simulink model "14_bus"  (R2024a)
settings: Solver=VariableStepAuto  StartTime=0.0  StopTime=1  RelTol=1e-3
undefined symbols (not defined in the file): D1, Delta
libraries: spsRMSLib x186, simulink_extras x171, spsThreePhaseVIMeasurementLib x94, spsThreePhaseBreakerLib x62, spsThreePhaseSeriesRLCBranchLib x20, spsThreePhaseSeriesRLCLoadLib x12, spsThreePhaseSourceLib x5, spsLoadFlowBusLib x5, spsStairGeneratorLib x5, spsThreePhaseTransformerTwoWindingsLib x5, spsThreePhaseFaultLib x5, sps_lib x1
(part 1 of 6)
settings Model: VariantFading=off  Creator=kedar  LastModifiedBy=kedar

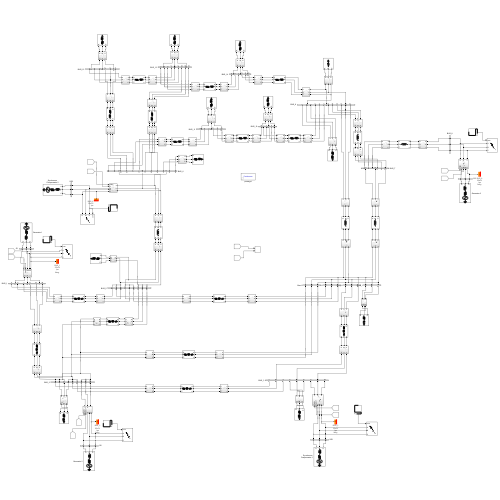
[thumbnail: Simulink's stored preview of the top-level diagram]
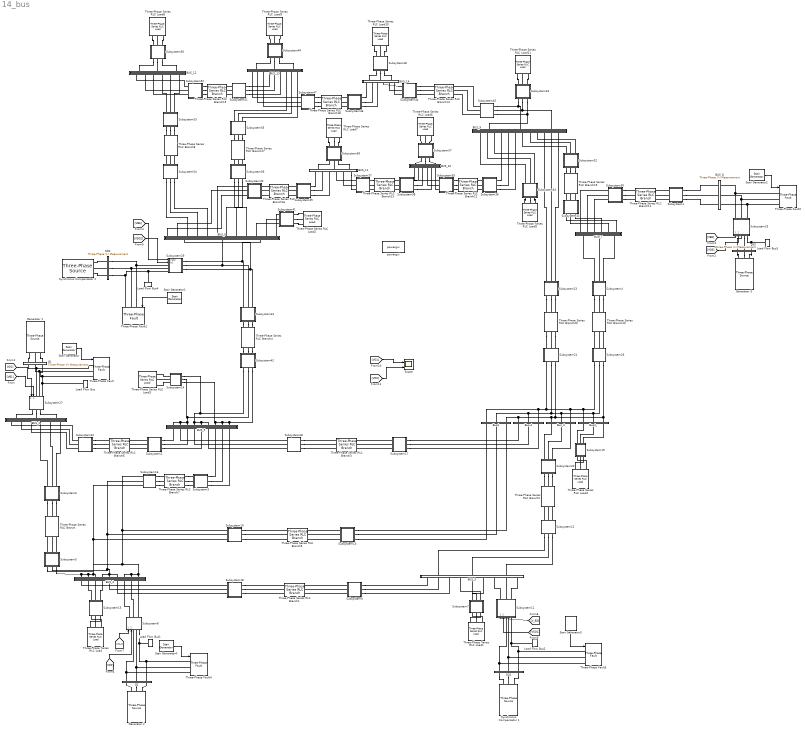
== system 14_bus ==
  BUS_1 : Subsystem
  BUS_10 : Subsystem
  BUS_11 : Subsystem
  BUS_12 : Subsystem
  BUS_13 : Subsystem
  BUS_14 : Subsystem
  BUS_2 : Subsystem
  BUS_3 : Subsystem
  BUS_5 : Subsystem
  BUS_6 : Subsystem
  BUS_7 : Subsystem
  BUS_8 : spsThreePhaseVIMeasurementLib/Three-Phase V-I Measurement  VoltageMeasurement=phase-to-ground  SetLabelV=on  LabelV=VB8  Vpu=off  VpuLL=off  CurrentMeasurement=yes  SetLabelI=on  LabelI=IB8  Ipu=off  Pbase=100e6  Vbase=0.95  OutputType=Complex  PhasorSimulation=off  PSBequivalent=0
  BUS_9 : Subsystem
  Bus-4 : spsThreePhaseVIMeasurementLib/Three-Phase V-I Measurement  VoltageMeasurement=phase-to-ground  SetLabelV=on  LabelV=VB4  Vpu=off  VpuLL=off  CurrentMeasurement=yes  SetLabelI=on  LabelI=IB4  Ipu=off  Pbase=100e6  Vbase=0.95  OutputType=Complex  PhasorSimulation=off  PSBequivalent=0
  Bus4 : spsThreePhaseVIMeasurementLib/Three-Phase V-I Measurement  VoltageMeasurement=phase-to-ground  SetLabelV=on  LabelV=VB_4  Vpu=off  VpuLL=off  CurrentMeasurement=yes  SetLabelI=on  LabelI=IB_4  Ipu=off  Pbase=100e6  Vbase=0.95  OutputType=Complex  PhasorSimulation=off  PSBequivalent=0
  Bus4_ : spsThreePhaseVIMeasurementLib/Three-Phase V-I Measurement  VoltageMeasurement=phase-to-ground  SetLabelV=on  LabelV=VB4_  Vpu=off  VpuLL=off  CurrentMeasurement=yes  SetLabelI=on  LabelI=IB4_  Ipu=off  Pbase=100e6  Vbase=0.95  OutputType=Complex  PhasorSimulation=off  PSBequivalent=0
  Bus_4 : spsThreePhaseVIMeasurementLib/Three-Phase V-I Measurement  VoltageMeasurement=phase-to-ground  SetLabelV=on  LabelV=V_B4  Vpu=off  VpuLL=off  CurrentMeasurement=yes  SetLabelI=on  LabelI=I_B4  Ipu=off  Pbase=100e6  Vbase=0.95  OutputType=Complex  PhasorSimulation=off  PSBequivalent=0
  G1 : spsThreePhaseVIMeasurementLib/Three-Phase V-I Measurement  VoltageMeasurement=phase-to-ground  SetLabelV=on  LabelV=VG1  Vpu=off  VpuLL=off  CurrentMeasurement=yes  SetLabelI=on  LabelI=IG1  Ipu=off  Pbase=100e6  Vbase=25e3  OutputType=Complex  PhasorSimulation=off  PSBequivalent=0
  G2 : spsThreePhaseVIMeasurementLib/Three-Phase V-I Measurement  VoltageMeasurement=phase-to-ground  SetLabelV=on  LabelV=VG2  Vpu=off  VpuLL=off  CurrentMeasurement=yes  SetLabelI=on  LabelI=IG2  Ipu=off  Pbase=100e6  Vbase=500e3  OutputType=Complex  PhasorSimulation=off  PSBequivalent=0
  G3 : spsThreePhaseVIMeasurementLib/Three-Phase V-I Measurement  VoltageMeasurement=phase-to-ground  SetLabelV=on  LabelV=VG3  Vpu=off  VpuLL=off  CurrentMeasurement=yes  SetLabelI=on  LabelI=IG3  Ipu=off  Pbase=100e6  Vbase=500e3  OutputType=Complex  PhasorSimulation=off  PSBequivalent=0
  Generator 1 : spsThreePhaseSourceLib/Three-Phase Source  InternalConnection=Yg  VoltagePhases=off  Voltage=25e3*1.060  PhaseAngle=0  Voltage_phases=[25e3 25e3 25e3]/sqrt(3)  PhaseAngles_phases=[0 -120 +120]  Frequency=50  NonIdealSource=on  SpecifyImpedance=on  Resistance=0.8929  Inductance=16.58e-3  ShortCircuitLevel=100e6  BaseVoltage=25e3  XRratio=7  BusType=swing  Pref=40e3  Qref=-40e3  Prefabc=[10e3, 10e3, 10e3]  Qrefabc=[0, 0, 0]  Qmin=-inf  Qmax=inf
  Generator 2 : spsThreePhaseSourceLib/Three-Phase Source  InternalConnection=Yg  VoltagePhases=off  Voltage=25e3*1.045  PhaseAngle=0  Voltage_phases=[25e3 25e3 25e3]/sqrt(3)  PhaseAngles_phases=[0 -120 +120]  Frequency=50  NonIdealSource=on  SpecifyImpedance=off  Resistance=0.8929  Inductance=16.58e-3  ShortCircuitLevel=100e6  BaseVoltage=25e3  XRratio=7  BusType=PV  Pref=232e3  Qref=0  Prefabc=[10e3, 10e3, 10e3]  Qrefabc=[0, 0, 0]  Qmin=-40e3  Qmax=50e3
  Generator 3 : spsThreePhaseSourceLib/Three-Phase Source  InternalConnection=Yg  VoltagePhases=off  Voltage=25e3*1.09  PhaseAngle=0  Voltage_phases=[25e3 25e3 25e3]/sqrt(3)  PhaseAngles_phases=[0 -120 +120]  Frequency=50  NonIdealSource=on  SpecifyImpedance=off  Resistance=0.8929  Inductance=16.58e-3  ShortCircuitLevel=100e6  BaseVoltage=25e3  XRratio=7  BusType=PQ  Pref=0  Qref=0  Prefabc=[10e3, 10e3, 10e3]  Qrefabc=[0, 0, 0]  Qmin=-6e3  Qmax=24e3
  Load Flow Bus : spsLoadFlowBusLib/Load Flow Bus  LConnTagsString=a  Phases=single  Connectors=on one side  ID=BUS_1  Vbase=25e3  Vref=1.06  Vangle=0  VLF=1  VLFb=1  VLFc=1  angleLF=0  angleLFb=0  angleLFc=0
  Load Flow Bus1 : spsLoadFlowBusLib/Load Flow Bus  LConnTagsString=a  Phases=single  Connectors=on one side  ID=BUS_2  Vbase=25e3  Vref=1.045  Vangle=0  VLF=1  VLFb=1  VLFc=1  angleLF=0  angleLFb=0  angleLFc=0
  Load Flow Bus2 : spsLoadFlowBusLib/Load Flow Bus  LConnTagsString=a  Phases=single  Connectors=on one side  ID=BUS_3  Vbase=25e3  Vref=1.01  Vangle=0  VLF=1  VLFb=1  VLFc=1  angleLF=0  angleLFb=0  angleLFc=0
  Load Flow Bus3 : spsLoadFlowBusLib/Load Flow Bus  LConnTagsString=a  Phases=single  Connectors=on one side  ID=BUS_8  Vbase=25e3  Vref=1.09  Vangle=0  VLF=1  VLFb=1  VLFc=1  angleLF=0  angleLFb=0  angleLFc=0
  Load Flow Bus4 : spsLoadFlowBusLib/Load Flow Bus  LConnTagsString=a  Phases=single  Connectors=on one side  ID=BUS_6  Vbase=25e3  Vref=1.07  Vangle=0  VLF=1  VLFb=1  VLFc=1  angleLF=0  angleLFb=0  angleLFc=0
  SG1 : spsThreePhaseVIMeasurementLib/Three-Phase V-I Measurement  VoltageMeasurement=phase-to-ground  SetLabelV=on  LabelV=VSG1  Vpu=off  VpuLL=off  CurrentMeasurement=yes  SetLabelI=on  LabelI=ISG1  Ipu=off  Pbase=100e6  Vbase=500e3  OutputType=Complex  PhasorSimulation=off  PSBequivalent=0
  SG2 : spsThreePhaseVIMeasurementLib/Three-Phase V-I Measurement  VoltageMeasurement=phase-to-ground  SetLabelV=on  LabelV=VSG2  Vpu=off  VpuLL=off  CurrentMeasurement=yes  SetLabelI=on  LabelI=ISG2  Ipu=off  Pbase=100e6  Vbase=500e3  OutputType=Complex  PhasorSimulation=off  PSBequivalent=0
  Scope : Scope  NumInputPorts=2
  Stair Generator{,1..4} (5 alike) : spsStairGeneratorLib/Stair Generator  t=[0, 1, 3, 3.5]  e=[1, -1, 2.5, 0]  Ts=0
  Subsystem1 : Subsystem
  Subsystem10 : Subsystem
  Subsystem11 : Subsystem
  Subsystem12 : Subsystem
  Subsystem13 : Subsystem
  Subsystem14 : Subsystem
  Subsystem15 : Subsystem
  Subsystem16 : Subsystem
  Subsystem17 : Subsystem
  Subsystem18 : Subsystem
  Subsystem19 : Subsystem
  Subsystem2 : Subsystem
  Subsystem20 : Subsystem
  Subsystem21 : Subsystem
  Subsystem22 : Subsystem
  Subsystem23 : Subsystem
  Subsystem25 : Subsystem
  Subsystem26 : Subsystem
  Subsystem27 : Subsystem
  Subsystem28 : Subsystem
  Subsystem29 : Subsystem
  Subsystem3 : Subsystem
  Subsystem30 : Subsystem
  Subsystem31 : Subsystem
  Subsystem32 : Subsystem
  Subsystem33 : Subsystem
  Subsystem34 : Subsystem
  Subsystem35 : Subsystem
  Subsystem36 : Subsystem
  Subsystem37 : Subsystem
  Subsystem38 : Subsystem
  Subsystem39 : Subsystem
  Subsystem4 : Subsystem
  Subsystem40 : Subsystem
  Subsystem41 : Subsystem
  Subsystem42 : Subsystem
  Subsystem43 : Subsystem
  Subsystem44 : Subsystem
  Subsystem45 : Subsystem
  Subsystem46 : Subsystem
  Subsystem47 : Subsystem
  Subsystem48 : Subsystem
  Subsystem49 : Subsystem
  Subsystem5 : Subsystem
  Subsystem50 : Subsystem
  Subsystem51 : Subsystem
  Subsystem52 : Subsystem
  Subsystem53 : Subsystem
  Subsystem54 : Subsystem
  Subsystem55 : Subsystem
  Subsystem56 : Subsystem
  Subsystem57 : Subsystem
  Subsystem58 : Subsystem
  Subsystem6 : Subsystem
  Subsystem7 : Subsystem
  Subsystem8 : Subsystem
  Subsystem9 : Subsystem
  Synchronus Compensator 1 : spsThreePhaseSourceLib/Three-Phase Source  InternalConnection=Yg  VoltagePhases=off  Voltage=25e3*1.01  PhaseAngle=0  Voltage_phases=[25e3 25e3 25e3]/sqrt(3)  PhaseAngles_phases=[0 -120 +120]  Frequency=50  NonIdealSource=on  SpecifyImpedance=off  Resistance=0.8929  Inductance=16.58e-3  ShortCircuitLevel=100e6  BaseVoltage=25e3  XRratio=7  BusType=PV  Pref=0  Qref=0  Prefabc=[10e3, 10e3, 10e3]  Qrefabc=[0, 0, 0]  Qmin=0  Qmax=50e3
  Synchronus Compensator 2 : spsThreePhaseSourceLib/Three-Phase Source  InternalConnection=Yg  VoltagePhases=off  Voltage=25e3*1.07  PhaseAngle=0  Voltage_phases=[25e3 25e3 25e3]/sqrt(3)  PhaseAngles_phases=[0 -120 +120]  Frequency=50  NonIdealSource=on  SpecifyImpedance=off  Resistance=0.8929  Inductance=16.58e-3  ShortCircuitLevel=100e6  BaseVoltage=25e3  XRratio=7  BusType=PV  Pref=0  Qref=0  Prefabc=[10e3, 10e3, 10e3]  Qrefabc=[0, 0, 0]  Qmin=-6e3  Qmax=24e3
  Three-Phase Series RLC Branch : spsThreePhaseSeriesRLCBranchLib/Three-Phase Series RLC Branch  LConnTagsString=A|B|C  RConnTagsString=A|B|C  BranchType=RLC  Resistance=1.94e-2  Inductance=0.05917/(2*pi*50)  Capacitance=1/0.0528/(2*pi*50)  Measurements=None
  Three-Phase Series RLC Branch1 : spsThreePhaseSeriesRLCBranchLib/Three-Phase Series RLC Branch  LConnTagsString=A|B|C  RConnTagsString=A|B|C  BranchType=RLC  Resistance=0.04699  Inductance=0.19797/(2*pi*50)  Capacitance=1/0.0374/(2*pi*50)  Measurements=None
  Three-Phase Series RLC Branch10 : spsThreePhaseSeriesRLCBranchLib/Three-Phase Series RLC Branch  LConnTagsString=A|B|C  RConnTagsString=A|B|C  BranchType=L  Resistance=0  Inductance=0.20912/(2*pi*50)  Capacitance=0  Measurements=None
  Three-Phase Series RLC Branch11 : spsThreePhaseSeriesRLCBranchLib/Three-Phase Series RLC Branch  LConnTagsString=A|B|C  RConnTagsString=A|B|C  BranchType=L  Resistance=0  Inductance=0.17615/(2*pi*50)  Capacitance=0  Measurements=None
  Three-Phase Series RLC Branch12 : spsThreePhaseSeriesRLCBranchLib/Three-Phase Series RLC Branch  LConnTagsString=A|B|C  RConnTagsString=A|B|C  BranchType=RL  Resistance=0.03181  Inductance=0.0845/(2*pi*50)  Capacitance=1e-6  Measurements=None
  Three-Phase Series RLC Branch13 : spsThreePhaseSeriesRLCBranchLib/Three-Phase Series RLC Branch  LConnTagsString=A|B|C  RConnTagsString=A|B|C  BranchType=RL  Resistance=0.08205  Inductance=0.19207/(2*pi*50)  Capacitance=1e-6  Measurements=None
  Three-Phase Series RLC Branch14 : spsThreePhaseSeriesRLCBranchLib/Three-Phase Series RLC Branch  LConnTagsString=A|B|C  RConnTagsString=A|B|C  BranchType=RL  Resistance=0.12711  Inductance=0.27038/(2*pi*50)  Capacitance=1e-6  Measurements=None
  Three-Phase Series RLC Branch15 : spsThreePhaseSeriesRLCBranchLib/Three-Phase Series RLC Branch  LConnTagsString=A|B|C  RConnTagsString=A|B|C  BranchType=RL  Resistance=0.22092  Inductance=0.19988/(2*pi*50)  Capacitance=1e-6  Measurements=None
  Three-Phase Series RLC Branch16 : spsThreePhaseSeriesRLCBranchLib/Three-Phase Series RLC Branch  LConnTagsString=A|B|C  RConnTagsString=A|B|C  BranchType=RL  Resistance=0.09498  Inductance=0.1989/(2*pi*50)  Capacitance=1e-6  Measurements=None
  Three-Phase Series RLC Branch17 : spsThreePhaseSeriesRLCBranchLib/Three-Phase Series RLC Branch  LConnTagsString=A|B|C  RConnTagsString=A|B|C  BranchType=RL  Resistance=0.06615  Inductance=0.13027/(2*pi*50)  Capacitance=1e-6  Measurements=None
  Three-Phase Series RLC Branch18 : spsThreePhaseSeriesRLCBranchLib/Three-Phase Series RLC Branch  LConnTagsString=A|B|C  RConnTagsString=A|B|C  BranchType=RL  Resistance=0.17093  Inductance=0.34802/(2*pi*50)  Capacitance=1e-6  Measurements=None
  Three-Phase Series RLC Branch19 : spsThreePhaseSeriesRLCBranchLib/Three-Phase Series RLC Branch  LConnTagsString=A|B|C  RConnTagsString=A|B|C  BranchType=L  Resistance=1  Inductance=0.11001/(2*pi*50)  Capacitance=1e-6  Measurements=None
  Three-Phase Series RLC Branch2 : spsThreePhaseSeriesRLCBranchLib/Three-Phase Series RLC Branch  LConnTagsString=A|B|C  RConnTagsString=A|B|C  BranchType=RLC  Resistance=0.06701  Inductance=0.17103/(2*pi*50)  Capacitance=1/0.0346/(2*pi*50)  Measurements=None
  Three-Phase Series RLC Branch20 : spsThreePhaseSeriesRLCBranchLib/Three-Phase Series RLC Branch  LConnTagsString=A|B|C  RConnTagsString=A|B|C  BranchType=L  Resistance=1  Inductance=0.55618/(2*pi*50)  Capacitance=1e-6  Measurements=None
  Three-Phase Series RLC Branch3 : spsThreePhaseSeriesRLCBranchLib/Three-Phase Series RLC Branch  LConnTagsString=A|B|C  RConnTagsString=A|B|C  BranchType=RLC  Resistance=0.01335  Inductance=0.04211/(2*pi*50)  Capacitance=1/0.0128/(2*pi*50)  Measurements=None
  Three-Phase Series RLC Branch4 : spsThreePhaseSeriesRLCBranchLib/Three-Phase Series RLC Branch  LConnTagsString=A|B|C  RConnTagsString=A|B|C  BranchType=L  Resistance=0  Inductance=0.25202/(2*pi*50)  Capacitance=0  Measurements=None
  Three-Phase Series RLC Branch5 : spsThreePhaseSeriesRLCBranchLib/Three-Phase Series RLC Branch  LConnTagsString=A|B|C  RConnTagsString=A|B|C  BranchType=RLC  Resistance=0.05811  Inductance=0.17632/(2*pi*50)  Capacitance=1/0.0492/(2*pi*50)  Measurements=None
  Three-Phase Series RLC Branch6 : spsThreePhaseSeriesRLCBranchLib/Three-Phase Series RLC Branch  LConnTagsString=A|B|C  RConnTagsString=A|B|C  BranchType=RLC  Resistance=0.05403  Inductance=0.22304/(2*pi*50)  Capacitance=1/0.0438/(2*pi*50)  Measurements=None
  Three-Phase Series RLC Branch7 : spsThreePhaseSeriesRLCBranchLib/Three-Phase Series RLC Branch  LConnTagsString=A|B|C  RConnTagsString=A|B|C  BranchType=RLC  Resistance=0.05695  Inductance=0.17388/(2*pi*50)  Capacitance=1/0.034/(2*pi*50)  Measurements=None
  Three-Phase Series RLC Branch8 : spsThreePhaseSeriesRLCBranchLib/Three-Phase Series RLC Branch  LConnTagsString=A|B|C  RConnTagsString=A|B|C  BranchType=RL  Resistance=0.12291  Inductance=0.25581/(2*pi*50)  Capacitance=1e-6  Measurements=None
  Three-Phase Series RLC Load : spsThreePhaseSeriesRLCLoadLib/Three-Phase Series RLC Load  LConnTagsString=A|B|C  Configuration=Y (grounded)  NominalVoltage=25e3*1.045  Vabc=[1e3 1e3 1e3]  Vabcp=[1e3 1e3 1e3]  NominalFrequency=50  UnbalancedPower=off  ActivePower=21.7e3  InductivePower=12.7e3  CapacitivePower=0  Pabc=[10e3 9e3 11e3]  QLabc=[100 90 110]  QCabc=[100 90 110]  Pabcp=[10e3 9e3 11e3]  QLabcp=[100 90 110]  QCabcp=[100 90 110]  Measurements=None  LoadType=constant Z
  Three-Phase Series RLC Load1 : spsThreePhaseSeriesRLCLoadLib/Three-Phase Series RLC Load  LConnTagsString=A|B|C  Configuration=Y (grounded)  NominalVoltage=25e3*1.01  Vabc=[1e3 1e3 1e3]  Vabcp=[1e3 1e3 1e3]  NominalFrequency=50  UnbalancedPower=off  ActivePower=94.2e3  InductivePower=19.1e3  CapacitivePower=0  Pabc=[10e3 9e3 11e3]  QLabc=[100 90 110]  QCabc=[100 90 110]  Pabcp=[10e3 9e3 11e3]  QLabcp=[100 90 110]  QCabcp=[100 90 110]  Measurements=None  LoadType=constant Z
  Three-Phase Series RLC Load10 : spsThreePhaseSeriesRLCLoadLib/Three-Phase Series RLC Load  LConnTagsString=A|B|C  Configuration=Y (grounded)  NominalVoltage=25e3  Vabc=[1e3 1e3 1e3]  Vabcp=[1e3 1e3 1e3]  NominalFrequency=50  UnbalancedPower=off  ActivePower=14.9e3  InductivePower=5e3  CapacitivePower=0  Pabc=[10e3 9e3 11e3]  QLabc=[100 90 110]  QCabc=[100 90 110]  Pabcp=[10e3 9e3 11e3]  QLabcp=[100 90 110]  QCabcp=[100 90 110]  Measurements=None  LoadType=constant Z
  Three-Phase Series RLC Load11 : spsThreePhaseSeriesRLCLoadLib/Three-Phase Series RLC Load  LConnTagsString=A|B|C  Configuration=Y (grounded)  NominalVoltage=25e3  Vabc=[1e3 1e3 1e3]  Vabcp=[1e3 1e3 1e3]  NominalFrequency=50  UnbalancedPower=off  ActivePower=0  InductivePower=0  CapacitivePower=25e6  Pabc=[10e3 9e3 11e3]  QLabc=[100 90 110]  QCabc=[100 90 110]  Pabcp=[10e3 9e3 11e3]  QLabcp=[100 90 110]  QCabcp=[100 90 110]  Measurements=None  LoadType=constant Z
  Three-Phase Series RLC Load2 : spsThreePhaseSeriesRLCLoadLib/Three-Phase Series RLC Load  LConnTagsString=A|B|C  Configuration=Y (grounded)  NominalVoltage=25e3*1.07  Vabc=[1e3 1e3 1e3]  Vabcp=[1e3 1e3 1e3]  NominalFrequency=50  UnbalancedPower=off  ActivePower=11.2e3  InductivePower=7.5e3  CapacitivePower=0  Pabc=[10e3 9e3 11e3]  QLabc=[100 90 110]  QCabc=[100 90 110]  Pabcp=[10e3 9e3 11e3]  QLabcp=[100 90 110]  QCabcp=[100 90 110]  Measurements=None  LoadType=constant Z
  Three-Phase Series RLC Load3 : spsThreePhaseSeriesRLCLoadLib/Three-Phase Series RLC Load  LConnTagsString=A|B|C  Configuration=Y (grounded)  NominalVoltage=25e3  Vabc=[1e3 1e3 1e3]  Vabcp=[1e3 1e3 1e3]  NominalFrequency=50  UnbalancedPower=off  ActivePower=7.6e3  InductivePower=1.6e3  CapacitivePower=0  Pabc=[10e3 9e3 11e3]  QLabc=[100 90 110]  QCabc=[100 90 110]  Pabcp=[10e3 9e3 11e3]  QLabcp=[100 90 110]  QCabcp=[100 90 110]  Measurements=None  LoadType=constant Z
  Three-Phase Series RLC Load4 : spsThreePhaseSeriesRLCLoadLib/Three-Phase Series RLC Load  LConnTagsString=A|B|C  Configuration=Y (grounded)  NominalVoltage=25e3  Vabc=[1e3 1e3 1e3]  Vabcp=[1e3 1e3 1e3]  NominalFrequency=50  UnbalancedPower=off  ActivePower=47.8e3  InductivePower=0  CapacitivePower=3.9e3  Pabc=[10e3 9e3 11e3]  QLabc=[100 90 110]  QCabc=[100 90 110]  Pabcp=[10e3 9e3 11e3]  QLabcp=[100 90 110]  QCabcp=[100 90 110]  Measurements=None  LoadType=constant Z
  Three-Phase Series RLC Load5 : spsThreePhaseSeriesRLCLoadLib/Three-Phase Series RLC Load  LConnTagsString=A|B|C  Configuration=Y (grounded)  NominalVoltage=25e3*1.07  Vabc=[1e3 1e3 1e3]  Vabcp=[1e3 1e3 1e3]  NominalFrequency=50  UnbalancedPower=off  ActivePower=29.5e3  InductivePower=16.6e3  CapacitivePower=0  Pabc=[10e3 9e3 11e3]  QLabc=[100 90 110]  QCabc=[100 90 110]  Pabcp=[10e3 9e3 11e3]  QLabcp=[100 90 110]  QCabcp=[100 90 110]  Measurements=None  LoadType=constant Z
  Three-Phase Series RLC Load6 : spsThreePhaseSeriesRLCLoadLib/Three-Phase Series RLC Load  LConnTagsString=A|B|C  Configuration=Y (grounded)  NominalVoltage=25e3*1.09  Vabc=[1e3 1e3 1e3]  Vabcp=[1e3 1e3 1e3]  NominalFrequency=50  UnbalancedPower=off  ActivePower=9e3  InductivePower=5.8e3  CapacitivePower=0  Pabc=[10e3 9e3 11e3]  QLabc=[100 90 110]  QCabc=[100 90 110]  Pabcp=[10e3 9e3 11e3]  QLabcp=[100 90 110]  QCabcp=[100 90 110]  Measurements=None  LoadType=constant Z
  Three-Phase Series RLC Load7 : spsThreePhaseSeriesRLCLoadLib/Three-Phase Series RLC Load  LConnTagsString=A|B|C  Configuration=Y (grounded)  NominalVoltage=25e3  Vabc=[1e3 1e3 1e3]  Vabcp=[1e3 1e3 1e3]  NominalFrequency=50  UnbalancedPower=off  ActivePower=3.5e3  InductivePower=1.8e3  CapacitivePower=0  Pabc=[10e3 9e3 11e3]  QLabc=[100 90 110]  QCabc=[100 90 110]  Pabcp=[10e3 9e3 11e3]  QLabcp=[100 90 110]  QCabcp=[100 90 110]  Measurements=None  LoadType=constant Z
  Three-Phase Series RLC Load8 : spsThreePhaseSeriesRLCLoadLib/Three-Phase Series RLC Load  LConnTagsString=A|B|C  Configuration=Y (grounded)  NominalVoltage=25e3  Vabc=[1e3 1e3 1e3]  Vabcp=[1e3 1e3 1e3]  NominalFrequency=50  UnbalancedPower=off  ActivePower=6.1e3  InductivePower=1.6e3  CapacitivePower=0  Pabc=[10e3 9e3 11e3]  QLabc=[100 90 110]  QCabc=[100 90 110]  Pabcp=[10e3 9e3 11e3]  QLabcp=[100 90 110]  QCabcp=[100 90 110]  Measurements=None  LoadType=constant Z
  Three-Phase Series RLC Load9 : spsThreePhaseSeriesRLCLoadLib/Three-Phase Series RLC Load  LConnTagsString=A|B|C  Configuration=Y (grounded)  NominalVoltage=25e3  Vabc=[1e3 1e3 1e3]  Vabcp=[1e3 1e3 1e3]  NominalFrequency=50  UnbalancedPower=off  ActivePower=13.8e3  InductivePower=5.8e3  CapacitivePower=0  Pabc=[10e3 9e3 11e3]  QLabc=[100 90 110]  QCabc=[100 90 110]  Pabcp=[10e3 9e3 11e3]  QLabcp=[100 90 110]  QCabcp=[100 90 110]  Measurements=None  LoadType=constant Z
  Three-Phase Fault{,1..4} (5 alike) : spsThreePhaseFaultLib/Three-Phase Fault  InitialStates=0  FaultA=off  FaultB=off  FaultC=off  GroundFault=off  SwitchTimes="[1/60  5/60]"  External=on  SwitchStatus=NaN  FaultResistance=0.001  GroundResistance=0.01  SnubberResistance=1e6  SnubberCapacitance=inf  Measurements=None
  powergui : sps_lib/powergui  Priority=1  SimulationMode=Continuous  SampleTime=50e-6  frequency=60  Iterations=50  frequencyindice=50  Pbase=100e6  ErrMax=1e-4  UnitsV=kV  UnitsW=MW  buscounter=0  FunctionMessages=off  echomessages=off  EnableUseOfTLC=off  CurrentSourceSwitches=off  DisableSnubberDevices=off  DisableRonSwitches=off  DisableVfSwitches=off  DisplayEquations=off  AutomaticDiscreteSolvers=off  SolverType=Tustin/Backward Euler (TBE)  Interpol=off  ExternalGateDelay=off  methode=off  Ts=100  x0status=blocks  SPID=on  SwTol=0  HookPort=off  NonlinearTolerance=1e-4  nMaxIteration=100  ContinueOnMaxIteration=off  RestoreLinks=warning  ResistiveCurrentMeasurement=off  Frange=[0:2:500]  Ylog=off  Xlog=on  ShowGrid=off  save=off  variable=ZData  structure=0  ZoomFFT=off  StartTime=0.0  cycles=1  DisplayStyle=1  fundamental=60  FreqAxis=off  MaxFrequency=1000  frequencyindicesteady=1  RmsSteady=1  display=off
  wires:
  [VB6] -> Subsystem29/1(Vabc)
  [VG2] -> Subsystem8/2(Vabc1)
  [VB1] -> Subsystem27/2(Vabc)
  [IG1] -> Subsystem27/1(In1)
  [VG3] -> Subsystem25/2(In2)
  [VB8] -> Subsystem25/1(Vabc)
  [VSG2] -> Subsystem29/2(In1)
  [VB_2] -> Subsystem8/1(Vabc)
  [V_B3] -> Subsystem11/1(Vabc)
  [VSG1] -> Subsystem11/2(Vabc1)
  [VG1] -> Scope/1
  [VG2] -> Scope/2
  Stair Generator/1 -> Three-Phase Fault/1
  Stair Generator1/1 -> Three-Phase Fault1/1
  Stair Generator2/1 -> Three-Phase Fault2/1
  Stair Generator3/1 -> Three-Phase Fault3/1
  Stair Generator4/1 -> Three-Phase Fault4/1
  connections:
  BUS_2/LConn9 -- BUS_2/LConn8 -- BUS_2/LConn7 -- Subsystem16/RConn1 -- Subsystem10/RConn1 -- Subsystem5/RConn1
  BUS_5/LConn6 -- BUS_5/LConn5 -- Subsystem14/RConn1 -- Subsystem42/RConn1 -- BUS_5/LConn4
  Bus4_/LConn3 -- Subsystem26/RConn3 -- Subsystem21/RConn3 -- Bus4/LConn3 -- Bus-4/LConn1 -- Bus_4/LConn1
  Bus4_/LConn2 -- Subsystem26/RConn2 -- Bus_4/LConn2 -- Subsystem21/RConn2 -- Bus4/LConn2 -- Bus-4/LConn2
  Bus4_/LConn1 -- Subsystem26/RConn1 -- Bus_4/LConn3 -- Subsystem21/RConn1 -- Bus4/LConn1 -- Bus-4/LConn3
  Subsystem33/RConn1 -- Subsystem45/RConn1 -- BUS_9/LConn2
  Subsystem33/RConn3 -- Subsystem45/RConn3 -- BUS_9/LConn1
  Subsystem33/RConn2 -- Subsystem45/RConn2 -- BUS_9/LConn3
  Subsystem42/RConn3 -- BUS_5/LConn9 -- BUS_5/LConn8 -- Subsystem14/RConn3 -- BUS_5/LConn7
  Subsystem14/RConn2 -- Subsystem42/RConn2 -- BUS_5/LConn2 -- BUS_5/LConn1 -- BUS_5/LConn3
  BUS_2/LConn6 -- Subsystem16/RConn2 -- Subsystem10/RConn2 -- Subsystem5/RConn2 -- BUS_2/LConn5 -- BUS_2/LConn4
  Subsystem43/RConn3 -- Subsystem29/RConn3 -- BUS_6/LConn1
  Subsystem43/RConn1 -- BUS_6/LConn3 -- Subsystem29/RConn1
  Subsystem43/RConn2 -- Subsystem29/RConn2 -- BUS_6/LConn2
  G1/LConn2 -- Generator 1/RConn2
  Generator 1/RConn1 -- G1/LConn1
  G2/LConn2 -- Generator 2/RConn2
  Generator 2/RConn1 -- G2/LConn1
  Generator 2/RConn3 -- G2/LConn3
  SG1/LConn1 -- Synchronus Compensator 1/RConn1
  SG1/LConn2 -- Synchronus Compensator 1/RConn2
  SG1/LConn3 -- Synchronus Compensator 1/RConn3
  G3/LConn2 -- Generator 3/RConn2
  G3/LConn1 -- Generator 3/RConn1
  G3/LConn3 -- Generator 3/RConn3
  Subsystem10/LConn1 -- Three-Phase Series RLC Branch5/LConn1
  Subsystem10/LConn2 -- Three-Phase Series RLC Branch5/LConn2
  Subsystem10/LConn3 -- Three-Phase Series RLC Branch5/LConn3
  Subsystem14/LConn1 -- Three-Phase Series RLC Load3/LConn1
  Subsystem14/LConn2 -- Three-Phase Series RLC Load3/LConn2
  Subsystem14/LConn3 -- Three-Phase Series RLC Load3/LConn3
  Subsystem5/RConn3 -- BUS_2/LConn1 -- BUS_2/LConn2 -- BUS_2/LConn3 -- Subsystem16/RConn3 -- Subsystem10/RConn3
  Subsystem3/RConn1 -- BUS_5/RConn7
  Subsystem3/RConn2 -- BUS_5/RConn8
  Subsystem3/RConn3 -- BUS_5/RConn9
  Three-Phase Series RLC Branch7/RConn1 -- Subsystem3/LConn1
  Three-Phase Series RLC Branch7/RConn2 -- Subsystem3/LConn2
  Three-Phase Series RLC Branch7/RConn3 -- Subsystem3/LConn3
  Subsystem16/LConn1 -- Three-Phase Series RLC Branch7/LConn1
  Subsystem16/LConn2 -- Three-Phase Series RLC Branch7/LConn2
  Subsystem16/LConn3 -- Three-Phase Series RLC Branch7/LConn3
  Subsystem15/RConn1 -- BUS_2/RConn2
  Subsystem15/RConn2 -- BUS_2/RConn3
  Subsystem15/RConn3 -- BUS_2/RConn4
  Subsystem8/RConn1 -- BUS_2/RConn7
  Subsystem8/RConn2 -- BUS_2/RConn8
  Subsystem8/RConn3 -- BUS_2/RConn9
  G2/RConn3 -- Subsystem8/LConn1 -- Three-Phase Fault4/LConn3
  G2/RConn2 -- Subsystem8/LConn2 -- Three-Phase Fault4/LConn2
  Subsystem8/LConn3 -- Load Flow Bus1/LConn1 -- G2/RConn1 -- Three-Phase Fault4/LConn1
  Subsystem7/RConn2 -- BUS_3/RConn5
  Subsystem11/RConn1 -- BUS_3/RConn7
  Subsystem11/RConn2 -- BUS_3/RConn8
  Subsystem11/RConn3 -- BUS_3/RConn9
  SG1/RConn3 -- Three-Phase Fault3/LConn3 -- Subsystem11/LConn1
  SG1/RConn2 -- Three-Phase Fault3/LConn2 -- Subsystem11/LConn2
  SG1/RConn1 -- Three-Phase Fault3/LConn1 -- Load Flow Bus2/LConn1 -- Subsystem11/LConn3
  Subsystem19/RConn1 -- Bus4_/RConn1
  Subsystem19/RConn2 -- Bus4_/RConn2
  Subsystem19/RConn3 -- Bus4_/RConn3
  Three-Phase Series RLC Branch20/RConn1 -- Subsystem21/LConn1
  Subsystem21/LConn2 -- Three-Phase Series RLC Branch20/RConn2
  Three-Phase Series RLC Branch20/RConn3 -- Subsystem21/LConn3
  Subsystem23/RConn1 -- BUS_9/RConn10
  Subsystem23/RConn2 -- BUS_9/RConn11
  Subsystem23/RConn3 -- BUS_9/RConn12
  Subsystem23/LConn2 -- Three-Phase Series RLC Branch20/LConn2
  Subsystem26/LConn1 -- Three-Phase Series RLC Branch10/RConn1
  Subsystem26/LConn2 -- Three-Phase Series RLC Branch10/RConn2
  Subsystem26/LConn3 -- Three-Phase Series RLC Branch10/RConn3
  Subsystem25/RConn1 -- BUS_8/RConn1 -- Three-Phase Fault2/LConn1
  Subsystem25/RConn2 -- BUS_8/RConn2 -- Three-Phase Fault2/LConn2
  Subsystem25/RConn3 -- Three-Phase Fault2/LConn3 -- BUS_8/RConn3
  Subsystem25/LConn1 -- G3/RConn1
  Subsystem25/LConn2 -- G3/RConn2
  Subsystem25/LConn3 -- Load Flow Bus3/LConn1 -- G3/RConn3
  G1/RConn1 -- Three-Phase Fault/LConn1 -- Subsystem27/LConn1
  G1/RConn2 -- Three-Phase Fault/LConn2 -- Subsystem27/LConn2
  G1/RConn3 -- Three-Phase Fault/LConn3 -- Load Flow Bus/LConn1 -- Subsystem27/LConn3
  Subsystem30/LConn1 -- Three-Phase Series RLC Branch11/LConn1
  Subsystem30/LConn2 -- Three-Phase Series RLC Branch11/LConn2
  Subsystem30/LConn3 -- Three-Phase Series RLC Branch11/LConn3
  Subsystem30/RConn1 -- BUS_7/RConn1
  Subsystem30/RConn2 -- BUS_7/RConn2
  Subsystem30/RConn3 -- BUS_7/RConn3
  Subsystem1/LConn1 -- Three-Phase Series RLC Branch11/RConn1
  Subsystem1/LConn2 -- Three-Phase Series RLC Branch11/RConn2
  Subsystem1/LConn3 -- Three-Phase Series RLC Branch11/RConn3
  Subsystem1/RConn2 -- BUS_8/LConn2
  Subsystem1/RConn1 -- BUS_8/LConn1
  Subsystem1/RConn3 -- BUS_8/LConn3
  Subsystem31/LConn1 -- Three-Phase Series RLC Branch19/RConn1
  Subsystem31/LConn2 -- Three-Phase Series RLC Branch19/RConn2
  Subsystem31/LConn3 -- Three-Phase Series RLC Branch19/RConn3
  Subsystem31/RConn2 -- BUS_7/RConn5
  Subsystem32/LConn2 -- Three-Phase Series RLC Branch19/LConn2
  Subsystem32/LConn1 -- Three-Phase Series RLC Branch19/LConn1
  Subsystem32/LConn3 -- Three-Phase Series RLC Branch19/LConn3
  Subsystem32/RConn1 -- BUS_9/RConn7
  Subsystem32/RConn2 -- BUS_9/RConn8
  Subsystem32/RConn3 -- BUS_9/RConn9
  Subsystem33/LConn2 -- Three-Phase Series RLC Load11/LConn2
  Three-Phase Series RLC Load11/LConn1 -- Subsystem33/LConn1
  Three-Phase Series RLC Load11/LConn3 -- Subsystem33/LConn3
  Subsystem34/LConn2 -- Three-Phase Series RLC Load5/LConn2
  Subsystem34/LConn1 -- Three-Phase Series RLC Load5/LConn1
  Subsystem34/LConn3 -- Three-Phase Series RLC Load5/LConn3
  Subsystem34/RConn1 -- BUS_9/RConn1
  Subsystem34/RConn2 -- BUS_9/RConn2
  Subsystem34/RConn3 -- BUS_9/RConn3
  Subsystem35/LConn1 -- Three-Phase Series RLC Branch12/LConn1
  Subsystem35/LConn2 -- Three-Phase Series RLC Branch12/LConn2
  Subsystem35/LConn3 -- Three-Phase Series RLC Branch12/LConn3
  Subsystem35/RConn1 -- BUS_10/RConn2
  Subsystem35/RConn2 -- BUS_10/RConn4
  Subsystem35/RConn3 -- BUS_10/RConn6
  Subsystem36/LConn1 -- Three-Phase Series RLC Branch12/RConn1
  Subsystem36/LConn2 -- Three-Phase Series RLC Branch12/RConn2
  Subsystem36/LConn3 -- Three-Phase Series RLC Branch12/RConn3
  Subsystem36/RConn1 -- BUS_9/RConn4
  Subsystem36/RConn2 -- BUS_9/RConn5
  Subsystem36/RConn3 -- BUS_9/RConn6
  Subsystem37/LConn1 -- Three-Phase Series RLC Branch13/LConn1
  Subsystem37/LConn2 -- Three-Phase Series RLC Branch13/LConn2
  Subsystem37/RConn1 -- BUS_11/RConn4
  Subsystem37/RConn2 -- BUS_11/RConn5
  BUS_11/RConn6 -- Subsystem37/RConn3
  Three-Phase Series RLC Branch13/LConn3 -- Subsystem37/LConn3
  Subsystem38/LConn1 -- Three-Phase Series RLC Branch13/RConn1
  Subsystem38/LConn2 -- Three-Phase Series RLC Branch13/RConn2
  Subsystem38/LConn3 -- Three-Phase Series RLC Branch13/RConn3
  Subsystem38/RConn1 -- BUS_10/RConn1
  Subsystem38/RConn2 -- BUS_10/RConn3
  Subsystem38/RConn3 -- BUS_10/RConn5
  Subsystem39/LConn1 -- Three-Phase Series RLC Branch16/RConn1
  Subsystem39/LConn2 -- Three-Phase Series RLC Branch16/RConn2
  Subsystem39/LConn3 -- Three-Phase Series RLC Branch16/RConn3
  Subsystem39/RConn1 -- BUS_11/RConn1
  Subsystem39/RConn2 -- BUS_11/RConn2
  Subsystem39/RConn3 -- BUS_11/RConn3
  Three-Phase Series RLC Branch16/LConn2 -- Subsystem40/LConn2
  Three-Phase Series RLC Branch16/LConn1 -- Subsystem40/LConn1
  Three-Phase Series RLC Branch16/LConn3 -- Subsystem40/LConn3
  Subsystem40/RConn2 -- BUS_6/RConn2
  Subsystem41/LConn2 -- Three-Phase Series RLC Load2/LConn2
  Subsystem41/LConn1 -- Three-Phase Series RLC Load2/LConn1
  Subsystem41/LConn3 -- Three-Phase Series RLC Load2/LConn3
  Subsystem41/RConn2 -- BUS_6/RConn11
  Three-Phase Series RLC Branch4/RConn2 -- Subsystem42/LConn2
  Three-Phase Series RLC Branch4/RConn1 -- Subsystem42/LConn1
  Three-Phase Series RLC Branch4/RConn3 -- Subsystem42/LConn3
  Subsystem43/LConn1 -- Three-Phase Series RLC Branch4/LConn1
  Subsystem43/LConn2 -- Three-Phase Series RLC Branch4/LConn2
  Subsystem43/LConn3 -- Three-Phase Series RLC Branch4/LConn3
  Subsystem44/LConn1 -- Three-Phase Series RLC Branch14/LConn1
  Subsystem44/LConn2 -- Three-Phase Series RLC Branch14/LConn2
  Subsystem44/LConn3 -- Three-Phase Series RLC Branch14/LConn3
  Subsystem44/RConn1 -- BUS_14/RConn4
  Subsystem44/RConn2 -- BUS_14/RConn5
  Subsystem44/RConn3 -- BUS_14/RConn6
  Subsystem45/LConn1 -- Three-Phase Series RLC Branch14/RConn1
  Subsystem45/LConn2 -- Three-Phase Series RLC Branch14/RConn2
  Subsystem45/LConn3 -- Three-Phase Series RLC Branch14/RConn3
  Subsystem46/LConn1 -- Three-Phase Series RLC Branch18/RConn1
  Subsystem46/LConn2 -- Three-Phase Series RLC Branch18/RConn2
  Subsystem46/LConn3 -- Three-Phase Series RLC Branch18/RConn3
  Subsystem46/RConn1 -- BUS_14/RConn1
  Subsystem46/RConn2 -- BUS_14/RConn2
  Subsystem46/RConn3 -- BUS_14/RConn3
  Subsystem47/LConn1 -- Three-Phase Series RLC Branch18/LConn1
  Subsystem47/LConn2 -- Three-Phase Series RLC Branch18/LConn2
  Subsystem47/LConn3 -- Three-Phase Series RLC Branch18/LConn3
  Subsystem47/RConn1 -- BUS_13/RConn1
  Subsystem47/RConn2 -- BUS_13/RConn2
  Subsystem47/RConn3 -- BUS_13/RConn3
  Subsystem48/LConn2 -- Three-Phase Series RLC Load10/LConn2
  Three-Phase Series RLC Load10/LConn1 -- Subsystem48/LConn1
  Three-Phase Series RLC Load10/LConn3 -- Subsystem48/LConn3
  Subsystem48/RConn1 -- BUS_14/LConn1
  Subsystem48/RConn2 -- BUS_14/LConn2
  Subsystem48/RConn3 -- BUS_14/LConn3
  Subsystem49/LConn1 -- Three-Phase Series RLC Load9/LConn1
  Subsystem49/LConn2 -- Three-Phase Series RLC Load9/LConn2
  Subsystem49/LConn3 -- Three-Phase Series RLC Load9/LConn3
  Subsystem50/LConn2 -- Three-Phase Series RLC Load8/LConn2
  Three-Phase Series RLC Load8/LConn1 -- Subsystem50/LConn1
  Three-Phase Series RLC Load8/LConn3 -- Subsystem50/LConn3
  Subsystem50/RConn1 -- BUS_12/LConn1
  Subsystem50/RConn2 -- BUS_12/LConn2
  Subsystem50/RConn3 -- BUS_12/LConn3
  Subsystem51/LConn1 -- Three-Phase Series RLC Branch15/RConn1
  Subsystem51/LConn2 -- Three-Phase Series RLC Branch15/RConn2
  Subsystem51/LConn3 -- Three-Phase Series RLC Branch15/RConn3
  Subsystem51/RConn1 -- BUS_13/RConn4
  Subsystem51/RConn2 -- BUS_13/RConn5
  Subsystem51/RConn3 -- BUS_13/RConn6
  Subsystem52/LConn1 -- Three-Phase Series RLC Branch15/LConn1
  Subsystem52/LConn2 -- Three-Phase Series RLC Branch15/LConn2
  Subsystem52/LConn3 -- Three-Phase Series RLC Branch15/LConn3
  Subsystem52/RConn1 -- BUS_12/RConn1
  Subsystem52/RConn2 -- BUS_12/RConn2
  Subsystem52/RConn3 -- BUS_12/RConn3
  Subsystem53/LConn1 -- Three-Phase Series RLC Branch8/LConn1
  Subsystem53/LConn2 -- Three-Phase Series RLC Branch8/LConn2
  Subsystem53/RConn2 -- BUS_12/RConn5
  Subsystem53/RConn1 -- BUS_12/RConn4
  Subsystem53/RConn3 -- BUS_12/RConn6
  Subsystem53/LConn3 -- Three-Phase Series RLC Branch8/LConn3
  Subsystem54/LConn1 -- Three-Phase Series RLC Branch8/RConn1
  Subsystem54/LConn2 -- Three-Phase Series RLC Branch8/RConn2
  Subsystem54/LConn3 -- Three-Phase Series RLC Branch8/RConn3
  Subsystem54/RConn1 -- BUS_6/RConn3
  Subsystem54/RConn2 -- BUS_6/RConn4
  Subsystem54/RConn3 -- BUS_6/RConn5
  Subsystem55/LConn3 -- Three-Phase Series RLC Branch17/LConn3
  Subsystem55/LConn2 -- Three-Phase Series RLC Branch17/LConn2
  Subsystem55/LConn1 -- Three-Phase Series RLC Branch17/LConn1
  Subsystem55/RConn1 -- BUS_13/RConn7
  Subsystem55/RConn2 -- BUS_13/RConn8
  Subsystem55/RConn3 -- BUS_13/RConn9
  Subsystem56/LConn1 -- Three-Phase Series RLC Branch17/RConn1
  Subsystem56/LConn2 -- Three-Phase Series RLC Branch17/RConn2
  Subsystem56/LConn3 -- Three-Phase Series RLC Branch17/RConn3
  Subsystem56/RConn2 -- BUS_6/RConn8
  Subsystem18/LConn1 -- Three-Phase Series RLC Branch1/LConn1
  Subsystem18/LConn2 -- Three-Phase Series RLC Branch1/LConn2
  Subsystem18/LConn3 -- Three-Phase Series RLC Branch1/LConn3
  Subsystem18/RConn1 -- BUS_2/RConn1
  Subsystem18/RConn2 -- BUS_2/RConn5
  Subsystem18/RConn3 -- BUS_2/RConn6
  Subsystem9/LConn1 -- Three-Phase Series RLC Branch1/RConn1
  Subsystem9/LConn2 -- Three-Phase Series RLC Branch1/RConn2
  Subsystem9/LConn3 -- Three-Phase Series RLC Branch1/RConn3
  Subsystem9/RConn1 -- BUS_3/RConn1
  Subsystem9/RConn2 -- BUS_3/RConn2
  Subsystem9/RConn3 -- BUS_3/RConn3
  Subsystem12/LConn1 -- Three-Phase Series RLC Branch2/RConn1
  Subsystem12/LConn2 -- Three-Phase Series RLC Branch2/RConn2
  Subsystem12/LConn3 -- Three-Phase Series RLC Branch2/RConn3
  Subsystem12/RConn1 -- BUS_3/LConn1
  Subsystem12/RConn2 -- BUS_3/LConn2
  Subsystem12/RConn3 -- BUS_3/LConn3
  Subsystem20/LConn1 -- Three-Phase Series RLC Branch2/LConn1
  Subsystem20/LConn2 -- Three-Phase Series RLC Branch2/LConn2
  Subsystem20/LConn3 -- Three-Phase Series RLC Branch2/LConn3
  Subsystem20/RConn1 -- Bus_4/RConn1
  Subsystem20/RConn2 -- Bus_4/RConn2
  Subsystem20/RConn3 -- Bus_4/RConn3
  Subsystem28/LConn1 -- Three-Phase Series RLC Branch3/LConn1
  Subsystem28/LConn2 -- Three-Phase Series RLC Branch3/LConn2
  Subsystem28/LConn3 -- Three-Phase Series RLC Branch3/LConn3
  Subsystem28/RConn1 -- BUS_5/RConn2
  Subsystem28/RConn2 -- BUS_5/RConn4
  Subsystem28/RConn3 -- BUS_5/RConn6
  Subsystem17/LConn1 -- Three-Phase Series RLC Branch3/RConn1
  Subsystem17/LConn2 -- Three-Phase Series RLC Branch3/RConn2
  Subsystem17/LConn3 -- Three-Phase Series RLC Branch3/RConn3
  Subsystem17/RConn1 -- Bus-4/RConn1
  Subsystem17/RConn2 -- Bus-4/RConn2
  Subsystem17/RConn3 -- Bus-4/RConn3
  Subsystem6/LConn1 -- Three-Phase Series RLC Branch/LConn1
  Subsystem6/LConn2 -- Three-Phase Series RLC Branch/LConn2
  Subsystem6/LConn3 -- Three-Phase Series RLC Branch/LConn3
  Subsystem5/LConn1 -- Three-Phase Series RLC Branch/RConn1
  Subsystem5/LConn2 -- Three-Phase Series RLC Branch/RConn2
  Subsystem5/LConn3 -- Three-Phase Series RLC Branch/RConn3
  Subsystem22/LConn1 -- Three-Phase Series RLC Branch6/LConn1
  Subsystem22/LConn2 -- Three-Phase Series RLC Branch6/LConn2
  Subsystem22/LConn3 -- Three-Phase Series RLC Branch6/LConn3
  Subsystem2/LConn1 -- Three-Phase Series RLC Branch6/RConn1
  Subsystem2/LConn2 -- Three-Phase Series RLC Branch6/RConn2
  Subsystem2/LConn3 -- Three-Phase Series RLC Branch6/RConn3
  Subsystem2/RConn1 -- BUS_5/RConn1
  Subsystem2/RConn2 -- BUS_5/RConn3
  Subsystem2/RConn3 -- BUS_5/RConn5
  SG2/LConn2 -- Synchronus Compensator 2/RConn2
  Synchronus Compensator 2/RConn1 -- SG2/LConn1
  Synchronus Compensator 2/RConn3 -- SG2/LConn3
  SG2/RConn1 -- Three-Phase Fault1/LConn1 -- Subsystem29/LConn1
  SG2/RConn2 -- Three-Phase Fault1/LConn2 -- Subsystem29/LConn2
  SG2/RConn3 -- Three-Phase Fault1/LConn3 -- Load Flow Bus4/LConn1 -- Subsystem29/LConn3
  Subsystem57/LConn2 -- Three-Phase Series RLC Load6/LConn2
  Three-Phase Series RLC Load6/LConn1 -- Subsystem57/LConn1
  Three-Phase Series RLC Load6/LConn3 -- Subsystem57/LConn3
  Subsystem57/RConn1 -- BUS_10/LConn1
  Subsystem57/RConn2 -- BUS_10/LConn2
  Subsystem57/RConn3 -- BUS_10/LConn3
  Three-Phase Series RLC Load7/LConn2 -- Subsystem58/LConn2
  Three-Phase Series RLC Load7/LConn1 -- Subsystem58/LConn1
  Three-Phase Series RLC Load7/LConn3 -- Subsystem58/LConn3
  Subsystem58/RConn1 -- BUS_11/LConn1
  BUS_11/LConn2 -- Subsystem58/RConn2
  Subsystem58/RConn3 -- BUS_11/LConn3
  Subsystem27/RConn1 -- BUS_1/LConn1
  Subsystem27/RConn2 -- BUS_1/LConn2
  Subsystem27/RConn3 -- BUS_1/LConn3
  Subsystem22/RConn1 -- BUS_1/RConn1
  Subsystem22/RConn2 -- BUS_1/RConn2
  Subsystem22/RConn3 -- BUS_1/RConn3
  Subsystem6/RConn1 -- BUS_1/RConn4
  Subsystem6/RConn2 -- BUS_1/RConn5
  Subsystem6/RConn3 -- BUS_1/RConn6
  Generator 1/RConn3 -- G1/LConn3
  Three-Phase Series RLC Load4/LConn1 -- Subsystem19/LConn3
  Three-Phase Series RLC Load4/LConn3 -- Subsystem19/LConn1
  Three-Phase Series RLC Load4/LConn2 -- Subsystem19/LConn2
  Three-Phase Series RLC Load1/LConn1 -- Subsystem7/LConn3
  Three-Phase Series RLC Load1/LConn3 -- Subsystem7/LConn1
  Three-Phase Series RLC Load1/LConn2 -- Subsystem7/LConn2
  Three-Phase Series RLC Load/LConn1 -- Subsystem15/LConn3
  Three-Phase Series RLC Load/LConn3 -- Subsystem15/LConn1
  Three-Phase Series RLC Load/LConn2 -- Subsystem15/LConn2
  Subsystem49/RConn2 -- BUS_13/LConn2
  Subsystem7/RConn3 -- BUS_3/RConn4
  Subsystem7/RConn1 -- BUS_3/RConn6
  Subsystem31/RConn3 -- BUS_7/RConn4
  Subsystem31/RConn1 -- BUS_7/RConn6
  Subsystem49/RConn1 -- BUS_13/LConn1
  Subsystem41/RConn1 -- BUS_6/RConn12
  Subsystem41/RConn3 -- BUS_6/RConn10
  Subsystem40/RConn1 -- BUS_6/RConn6
  Subsystem40/RConn3 -- BUS_6/RConn1
  Subsystem13/LConn1 -- Three-Phase Series RLC Branch5/RConn1
  Subsystem13/LConn2 -- Three-Phase Series RLC Branch5/RConn2
  Subsystem13/LConn3 -- Three-Phase Series RLC Branch5/RConn3
  Subsystem13/RConn1 -- Bus4/RConn3
  Subsystem13/RConn2 -- Bus4/RConn2
  Subsystem13/RConn3 -- Bus4/RConn1
  Subsystem56/RConn3 -- BUS_6/RConn7
  Subsystem56/RConn1 -- BUS_6/RConn9
  Subsystem4/LConn2 -- Three-Phase Series RLC Branch10/LConn2
  Subsystem4/LConn1 -- Three-Phase Series RLC Branch10/LConn1
  Subsystem4/LConn3 -- Three-Phase Series RLC Branch10/LConn3
  Subsystem23/LConn1 -- Three-Phase Series RLC Branch20/LConn1
  Subsystem23/LConn3 -- Three-Phase Series RLC Branch20/LConn3
  Subsystem49/RConn3 -- BUS_13/LConn3
  Subsystem4/RConn1 -- BUS_7/LConn1
  BUS_7/LConn2 -- Subsystem4/RConn2
  Subsystem4/RConn3 -- BUS_7/LConn3

== system 14_bus/BUS_1 ==
  Bus-1 : spsThreePhaseVIMeasurementLib/Three-Phase V-I Measurement  VoltageMeasurement=phase-to-ground  SetLabelV=on  LabelV=VB1  Vpu=off  VpuLL=off  CurrentMeasurement=yes  SetLabelI=on  LabelI=IB1  Ipu=off  Pbase=100e6  Vbase=0.95  OutputType=Complex  PhasorSimulation=off  PSBequivalent=0
  Bus1 : spsThreePhaseVIMeasurementLib/Three-Phase V-I Measurement  VoltageMeasurement=no  SetLabelV=off  LabelV=Vabc  Vpu=on  VpuLL=off  CurrentMeasurement=no  SetLabelI=off  LabelI=Iabc  Ipu=on  Pbase=100e6  Vbase=0.95  OutputType=Complex  PhasorSimulation=off  PSBequivalent=0
  C : PMIOPort  Side=Left
  B : PMIOPort  Port=2  Side=Left
  C1 : PMIOPort  Port=3  Side=Left
  a : PMIOPort  Port=4  Side=Right
  b : PMIOPort  Port=5  Side=Right
  c : PMIOPort  Port=6  Side=Right
  c1 : PMIOPort  Port=7  Side=Right
  b1 : PMIOPort  Port=8  Side=Right
  a1 : PMIOPort  Port=9  Side=Right
  connections:
  Bus-1/LConn1 -- C1/RConn1 -- Bus1/LConn3
  a1/RConn1 -- Bus-1/RConn1
  c/RConn1 -- Bus1/RConn3
  Bus1/LConn2 -- B/RConn1 -- Bus-1/LConn2
  b1/RConn1 -- Bus-1/RConn2
  Bus1/LConn1 -- C/RConn1 -- Bus-1/LConn3
  b/RConn1 -- Bus1/RConn2
  a/RConn1 -- Bus1/RConn1
  c1/RConn1 -- Bus-1/RConn3

== system 14_bus/BUS_10 ==
  Bus-10 : spsThreePhaseVIMeasurementLib/Three-Phase V-I Measurement  VoltageMeasurement=phase-to-ground  SetLabelV=on  LabelV=VB10  Vpu=off  VpuLL=off  CurrentMeasurement=yes  SetLabelI=on  LabelI=IB10  Ipu=off  Pbase=100e6  Vbase=0.95  OutputType=Complex  PhasorSimulation=off  PSBequivalent=0
  Bus10 : spsThreePhaseVIMeasurementLib/Three-Phase V-I Measurement  VoltageMeasurement=phase-to-ground  SetLabelV=on  LabelV=VB_10  Vpu=off  VpuLL=off  CurrentMeasurement=yes  SetLabelI=on  LabelI=IB_10  Ipu=off  Pbase=100e6  Vbase=0.95  OutputType=Complex  PhasorSimulation=off  PSBequivalent=0
  A : PMIOPort  Side=Left
  B : PMIOPort  Port=2  Side=Left
  C : PMIOPort  Port=3  Side=Left
  a : PMIOPort  Port=4  Side=Right
  c : PMIOPort  Port=5  Side=Right
  b : PMIOPort  Port=6  Side=Right
  b1 : PMIOPort  Port=7  Side=Right
  c1 : PMIOPort  Port=8  Side=Right
  a1 : PMIOPort  Port=9  Side=Right
  connections:
  Bus10/LConn1 -- C/RConn1 -- Bus-10/LConn3
  Bus-10/LConn2 -- B/RConn1 -- Bus10/LConn2
  Bus10/LConn3 -- A/RConn1 -- Bus-10/LConn1
  Bus10/RConn2 -- b1/RConn1
  c1/RConn1 -- Bus-10/RConn3
  Bus10/RConn3 -- c/RConn1
  Bus10/RConn1 -- a1/RConn1
  b/RConn1 -- Bus-10/RConn2
  a/RConn1 -- Bus-10/RConn1

== system 14_bus/BUS_11 ==
  Bus-11 : spsThreePhaseVIMeasurementLib/Three-Phase V-I Measurement  VoltageMeasurement=phase-to-ground  SetLabelV=on  LabelV=VB11  Vpu=off  VpuLL=off  CurrentMeasurement=yes  SetLabelI=on  LabelI=IB11  Ipu=off  Pbase=100e6  Vbase=0.95  OutputType=Complex  PhasorSimulation=off  PSBequivalent=0
  Bus11 : spsThreePhaseVIMeasurementLib/Three-Phase V-I Measurement  VoltageMeasurement=phase-to-ground  SetLabelV=on  LabelV=VB_11  Vpu=off  VpuLL=off  CurrentMeasurement=yes  SetLabelI=on  LabelI=IB_11  Ipu=off  Pbase=100e6  Vbase=0.95  OutputType=Complex  PhasorSimulation=off  PSBequivalent=0
  A : PMIOPort  Side=Left
  B : PMIOPort  Port=2  Side=Left
  A1 : PMIOPort  Port=3  Side=Left
  a : PMIOPort  Port=4  Side=Right
  b : PMIOPort  Port=5  Side=Right
  c : PMIOPort  Port=6  Side=Right
  c1 : PMIOPort  Port=7  Side=Right
  b1 : PMIOPort  Port=8  Side=Right
  a1 : PMIOPort  Port=9  Side=Right
  connections:
  b1/RConn1 -- Bus11/RConn2
  Bus-11/LConn3 -- A1/RConn1 -- Bus11/LConn1
  a/RConn1 -- Bus-11/RConn1
  b/RConn1 -- Bus-11/RConn2
  c1/RConn1 -- Bus11/RConn3
  Bus11/LConn2 -- B/RConn1 -- Bus-11/LConn2
  a1/RConn1 -- Bus11/RConn1
  Bus11/LConn3 -- A/RConn1 -- Bus-11/LConn1
  c/RConn1 -- Bus-11/RConn3

== system 14_bus/BUS_12 ==
  Bus-12 : spsThreePhaseVIMeasurementLib/Three-Phase V-I Measurement  VoltageMeasurement=phase-to-ground  SetLabelV=on  LabelV=VB12  Vpu=off  VpuLL=off  CurrentMeasurement=yes  SetLabelI=on  LabelI=IB12  Ipu=off  Pbase=100e6  Vbase=0.95  OutputType=Complex  PhasorSimulation=off  PSBequivalent=0
  Bus12 : spsThreePhaseVIMeasurementLib/Three-Phase V-I Measurement  VoltageMeasurement=phase-to-ground  SetLabelV=on  LabelV=VB_12  Vpu=off  VpuLL=off  CurrentMeasurement=yes  SetLabelI=on  LabelI=IB_12  Ipu=off  Pbase=100e6  Vbase=0.95  OutputType=Complex  PhasorSimulation=off  PSBequivalent=0
  A : PMIOPort  Side=Left
  B : PMIOPort  Port=2  Side=Left
  A1 : PMIOPort  Port=3  Side=Left
  c : PMIOPort  Port=4  Side=Right
  b : PMIOPort  Port=5  Side=Right
  a : PMIOPort  Port=6  Side=Right
  a1 : PMIOPort  Port=7  Side=Right
  b1 : PMIOPort  Port=8  Side=Right
  c1 : PMIOPort  Port=9  Side=Right
  connections:
  c1/RConn1 -- Bus-12/RConn3
  Bus12/LConn3 -- A/RConn1 -- Bus-12/LConn1
  a1/RConn1 -- Bus-12/RConn1
  Bus-12/LConn3 -- A1/RConn1 -- Bus12/LConn1
  b1/RConn1 -- Bus-12/RConn2
  Bus12/LConn2 -- B/RConn1 -- Bus-12/LConn2
  a/RConn1 -- Bus12/RConn1
  b/RConn1 -- Bus12/RConn2
  c/RConn1 -- Bus12/RConn3

== system 14_bus/BUS_13 ==
  Bus-13 : spsThreePhaseVIMeasurementLib/Three-Phase V-I Measurement  VoltageMeasurement=phase-to-ground  SetLabelV=on  LabelV=VB13  Vpu=off  VpuLL=off  CurrentMeasurement=yes  SetLabelI=on  LabelI=IB13  Ipu=off  Pbase=100e6  Vbase=0.95  OutputType=Complex  PhasorSimulation=off  PSBequivalent=0
  Bus13 : spsThreePhaseVIMeasurementLib/Three-Phase V-I Measurement  VoltageMeasurement=phase-to-ground  SetLabelV=on  LabelV=VB_13  Vpu=off  VpuLL=off  CurrentMeasurement=yes  SetLabelI=on  LabelI=IB_13  Ipu=off  Pbase=100e6  Vbase=0.95  OutputType=Complex  PhasorSimulation=off  PSBequivalent=0
  Bus_13 : spsThreePhaseVIMeasurementLib/Three-Phase V-I Measurement  VoltageMeasurement=phase-to-ground  SetLabelV=on  LabelV=V_B13  Vpu=off  VpuLL=off  CurrentMeasurement=yes  SetLabelI=on  LabelI=I_B13  Ipu=off  Pbase=100e6  Vbase=0.95  OutputType=Complex  PhasorSimulation=off  PSBequivalent=0
  C : PMIOPort  Side=Left
  B : PMIOPort  Port=2  Side=Left
  A : PMIOPort  Port=3  Side=Left
  c : PMIOPort  Port=4  Side=Right
  b : PMIOPort  Port=5  Side=Right
  a : PMIOPort  Port=6  Side=Right
  c1 : PMIOPort  Port=7  Side=Right
  b1 : PMIOPort  Port=8  Side=Right
  a1 : PMIOPort  Port=9  Side=Right
  a2 : PMIOPort  Port=10  Side=Right
  b2 : PMIOPort  Port=11  Side=Right
  c2 : PMIOPort  Port=12  Side=Right
  connections:
  Bus_13/LConn1 -- A/RConn1 -- Bus-13/LConn1 -- Bus13/LConn3
  Bus_13/LConn3 -- C/RConn1 -- Bus13/LConn1 -- Bus-13/LConn3
  a2/RConn1 -- Bus13/RConn1
  Bus-13/LConn2 -- B/RConn1 -- Bus_13/LConn2 -- Bus13/LConn2
  c1/RConn1 -- Bus-13/RConn3
  a1/RConn1 -- Bus-13/RConn1
  c/RConn1 -- Bus_13/RConn3
  b/RConn1 -- Bus_13/RConn2
  c2/RConn1 -- Bus13/RConn3
  Bus_13/RConn1 -- a/RConn1
  b1/RConn1 -- Bus-13/RConn2
  b2/RConn1 -- Bus13/RConn2

== system 14_bus/BUS_14 ==
  Bus-14 : spsThreePhaseVIMeasurementLib/Three-Phase V-I Measurement  VoltageMeasurement=phase-to-ground  SetLabelV=on  LabelV=VB14  Vpu=off  VpuLL=off  CurrentMeasurement=yes  SetLabelI=on  LabelI=IB14  Ipu=off  Pbase=100e6  Vbase=0.95  OutputType=Complex  PhasorSimulation=off  PSBequivalent=0
  Bus14 : spsThreePhaseVIMeasurementLib/Three-Phase V-I Measurement  VoltageMeasurement=phase-to-ground  SetLabelV=on  LabelV=VB_14  Vpu=off  VpuLL=off  CurrentMeasurement=yes  SetLabelI=on  LabelI=IB_14  Ipu=off  Pbase=100e6  Vbase=0.95  OutputType=Complex  PhasorSimulation=off  PSBequivalent=0
  A : PMIOPort  Side=Left
  B : PMIOPort  Port=2  Side=Left
  A1 : PMIOPort  Port=3  Side=Left
  a : PMIOPort  Port=4  Side=Right
  b : PMIOPort  Port=5  Side=Right
  c : PMIOPort  Port=6  Side=Right
  c1 : PMIOPort  Port=7  Side=Right
  b1 : PMIOPort  Port=8  Side=Right
  a1 : PMIOPort  Port=9  Side=Right
  connections:
  Bus14/RConn2 -- b1/RConn1
  a/RConn1 -- Bus-14/RConn1
  Bus14/LConn3 -- A/RConn1 -- Bus-14/LConn1
  Bus14/LConn2 -- B/RConn1 -- Bus-14/LConn2
  c/RConn1 -- Bus-14/RConn3
  Bus-14/LConn3 -- A1/RConn1 -- Bus14/LConn1
  b/RConn1 -- Bus-14/RConn2
  Bus14/RConn1 -- a1/RConn1
  Bus14/RConn3 -- c1/RConn1

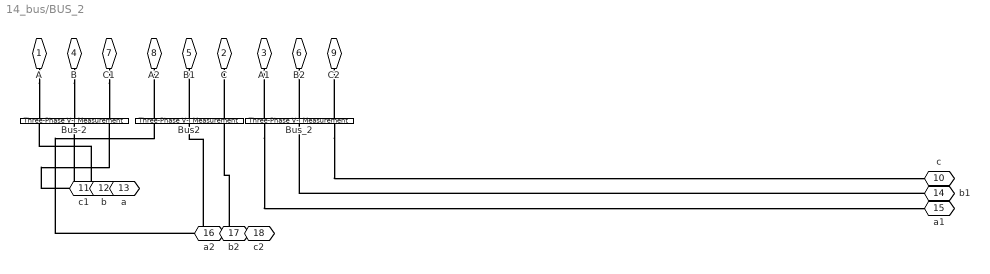
== system 14_bus/BUS_2 ==
  Bus-2 : spsThreePhaseVIMeasurementLib/Three-Phase V-I Measurement  VoltageMeasurement=phase-to-ground  SetLabelV=on  LabelV=VB2  Vpu=off  VpuLL=off  CurrentMeasurement=yes  SetLabelI=on  LabelI=IB2  Ipu=off  Pbase=100e6  Vbase=0.95  OutputType=Complex  PhasorSimulation=off  PSBequivalent=0
  Bus2 : spsThreePhaseVIMeasurementLib/Three-Phase V-I Measurement  VoltageMeasurement=phase-to-ground  SetLabelV=on  LabelV=VB_2  Vpu=off  VpuLL=off  CurrentMeasurement=yes  SetLabelI=on  LabelI=IB_2  Ipu=off  Pbase=100e6  Vbase=0.95  OutputType=Complex  PhasorSimulation=off  PSBequivalent=0
  Bus_2 : spsThreePhaseVIMeasurementLib/Three-Phase V-I Measurement  VoltageMeasurement=phase-to-ground  SetLabelV=on  LabelV=V_B2  Vpu=off  VpuLL=off  CurrentMeasurement=yes  SetLabelI=on  LabelI=I_B2  Ipu=off  Pbase=100e6  Vbase=0.95  OutputType=Complex  PhasorSimulation=off  PSBequivalent=0
  A : PMIOPort  Side=Left
  C : PMIOPort  Port=2  Side=Left
  A1 : PMIOPort  Port=3  Side=Left
  B : PMIOPort  Port=4  Side=Left
  B1 : PMIOPort  Port=5  Side=Left
  B2 : PMIOPort  Port=6  Side=Left
  C1 : PMIOPort  Port=7  Side=Left
  A2 : PMIOPort  Port=8  Side=Left
  C2 : PMIOPort  Port=9  Side=Left
  c : PMIOPort  Port=10  Side=Right
  c1 : PMIOPort  Port=11  Side=Right
  b : PMIOPort  Port=12  Side=Right
  a : PMIOPort  Port=13  Side=Right
  b1 : PMIOPort  Port=14  Side=Right
  a1 : PMIOPort  Port=15  Side=Right
  a2 : PMIOPort  Port=16  Side=Right
  b2 : PMIOPort  Port=17  Side=Right
  c2 : PMIOPort  Port=18  Side=Right
  connections:
  c1/RConn1 -- Bus-2/RConn3
  B/RConn1 -- Bus-2/LConn2
  Bus2/LConn2 -- B1/RConn1
  c2/RConn1 -- Bus2/RConn3
  a2/RConn1 -- Bus2/RConn1
  Bus_2/RConn3 -- c/RConn1
  Bus2/LConn1 -- A2/RConn1
  b/RConn1 -- Bus-2/RConn2
  Bus_2/LConn2 -- B2/RConn1
  Bus2/LConn3 -- C/RConn1
  Bus_2/RConn1 -- a1/RConn1
  Bus_2/LConn3 -- C2/RConn1
  C1/RConn1 -- Bus-2/LConn3
  A/RConn1 -- Bus-2/LConn1
  Bus_2/LConn1 -- A1/RConn1
  b2/RConn1 -- Bus2/RConn2
  a/RConn1 -- Bus-2/RConn1
  b1/RConn1 -- Bus_2/RConn2
